simulink model "sample_sys"  (R2022a)
settings: Solver=FixedStepDiscrete  StartTime=0.0  StopTime=T_final  FixedStep=T_sample  RelTol=1e-3
values from neighbouring files (symbols this model uses):
  A_bar_d = [0.9950 0.0998 ... (first row only)    [Run_model.m]    (also in prepare_trajectory_data.m)
  B_bar_d = [0.1 ... (first row only)    [Run_model.m]    (also in prepare_trajectory_data.m)
  C_obsv_d = [-0.48244804282  -0.463279461508; 0.0144227342104  -0.230554726046; 0.244765695792  -0.329721244669; 0.487562807757  0.730038636795; 0.684075320502  -0.191202440855; 0.0380669049625  0.232348391545]    [C_obsv_d.mat]    (also in sys_generation_WDS.m = C_obsv)
  D_obsv_d = zeros(n_meas,n_int)    [Run_model.m]    (also in prepare_trajectory_data.m; sys_generation_WDS.m = D_obsv)
  x0 = [7;7]    [Run_model.m]    (also in prepare_trajectory_data.m; test.m = rand(n_states,1))
settings Model: Creator=Abelb  LastModifiedBy=digitalstorm
settings DebuggingCC: UnconnectedInputMsg=warning  UnconnectedOutputMsg=warning  UnconnectedLineMsg=warning
settings RTWCC: DLArmComputeVersion=19.05

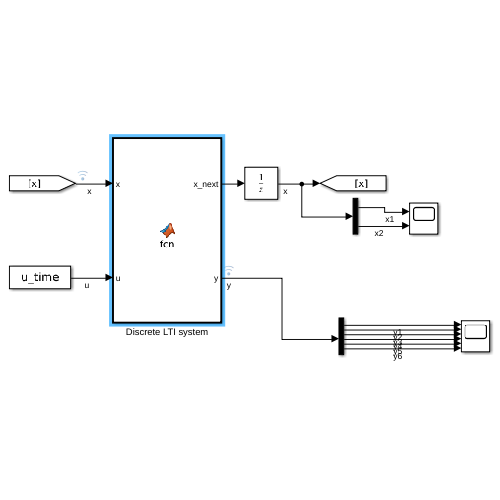
[thumbnail: Simulink's stored preview of the top-level diagram]
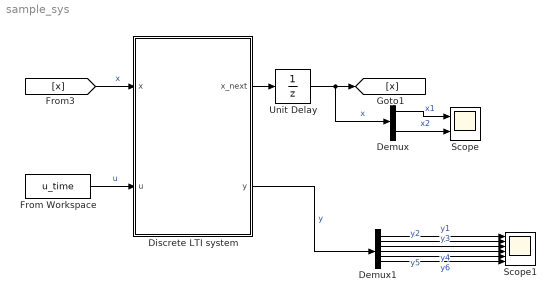
== system sample_sys ==
  Demux : Demux  Outputs=2
  Demux1 : Demux  Outputs=6
  Discrete LTI system : MATLAB Function  TreatAsAtomicUnit=on
  From Workspace : FromWorkspace  VariableName=u_time
  Scope : Scope  NumInputPorts=2
  Scope1 : Scope  NumInputPorts=6
  Unit Delay : UnitDelay  InitialCondition=x0  SampleTime=-1  HasFrameUpgradeWarning=on
  wires:
  Discrete LTI system/1(x_next) -> Unit Delay/1
  From Workspace/1 -> Discrete LTI system/2(u)  "u"
  Unit Delay/1 -> Demux/1, [x]  "x"
  [x] -> Discrete LTI system/1(x)  "x"
  Discrete LTI system/2(y) -> Demux1/1  "y"
  Demux/1 -> Scope/1  "x1"
  Demux/2 -> Scope/2  "x2"
  Demux1/1 -> Scope1/1  "y1"
  Demux1/2 -> Scope1/2  "y2"
  Demux1/3 -> Scope1/3  "y3"
  Demux1/4 -> Scope1/4  "y4"
  Demux1/5 -> Scope1/5  "y5"
  Demux1/6 -> Scope1/6  "y6"

== matlab function sample_sys/Discrete LTI system ==
  data: x input; x_next output; u input; y output; A_bar_d parameter; C_obsv_d parameter; B_bar_d parameter; D_obsv_d parameter
function [x_next,y] = fcn(x,u,A_bar_d,C_obsv_d,B_bar_d,D_obsv_d)
% Discrete state-space model for system

x_next = A_bar_d*x + B_bar_d*u;

y = C_obsv_d*x + D_obsv_d*u;
